simulink model "PassengerCar"  (R2019b)
settings: Solver=ode1  StartTime=0  StopTime=25  FixedStep=1.0000000000000000e-003  RelTol=1e-3
InitFcn:
  | sampleTime = str2double(get_param(bdroot, 'FixedStep'));
undefined symbols (not defined in the file or in its folder): AccPedalPos, BrakePedalPos, BrakeSwitch, DiscIntNeverNeededParam, DYNA4, EngSpd, IgnitionSwitch, InitialGear, InitialSpeed, IntendedEngTrq, LeftIndicator, MainBrakePress, MaxGear, MDL, MinGear, RefAcc, RefLane, RefLatPos, RefPath, RefPathCurv, RefSpd, RefSpdPreview, RefSpdRetrospect, RightIndicator, SteeringWheelAng, SteeringWheelTrq, UserDefinedRefValue, vm_const
libraries: UtilitiesLibrary x31, simulink x18, WheelSystemModules x13, LongitudinalControllerModules x13, LateralControllerModules x7, AnimationBusselectorModules x5, EnvironmentModules x5, BasicEngineControlModules x5, MiscellaneousControlModules x5, Animation3Modules x4, AuxiliariesModules x4, TireModules x4
(part 29 of 39)

== system PassengerCar/Vehicle/BrakeSystem/BrakeSystemControlUnit/BasicElectronicStabilityControl/BasicAntiLockBrakeControl ==
  ABSSwitchFromVehicleControl[0;1] : Inport
  RequiredWheelBrakePressures[Pa] : Inport  Port=2
  Vel_wrt_WorldSys(VehSys)[m/s] : Inport  Description=Maximum brake pressure  Port=3
  FrontLeftWheelLongSpd(ContactSys)[m/s] : Inport  Port=4
  FrontLeftWheelRotSpd[rad/s] : Inport  Port=5
  FrontLeftWheelRotAcc[rad/s**2] : Inport  Port=6
  FrontLeftTireDynamicRadius[m] : Inport  Port=7
  FrontRightWheelLongSpd(ContactSys)[m/s] : Inport  Port=8
  FrontRightWheelRotSpd[rad/s] : Inport  Port=9
  FrontRightWheelRotAcc[rad/s**2] : Inport  Port=10
  FrontRightTireDynamicRadius[m] : Inport  Port=11
  RearLeftWheelLongSpd(ContactSys)[m/s] : Inport  Port=12
  RearLeftWheelRotSpd[rad/s] : Inport  Port=13
  RearLeftWheelRotAcc[rad/s**2] : Inport  Port=14
  RearLeftTireDynamicRadius[m] : Inport  Port=15
  RearRightWheelLongSpd(ContactSys)[m/s] : Inport  Port=16
  RearRightWheelRotSpd[rad/s] : Inport  Port=17
  RearRightWheelRotAcc[rad/s**2] : Inport  Port=18
  RearRightTireDynamicRadius[m] : Inport  Port=19
  MaxMainBrakePress[Pa] : Inport  Description=Maximum brake pressure  Port=20
  AntiLockBrakeSystemOutput : Subsystem  Tag=TESIS DYNAware Interface Block  mask{NeedsUpdate=off, SignalInfo=|}
      mask SignalInfo=|
      | {
      |   "Version": "4.6",
      |   "MuxedOutputBusName": "AntiLockBrakeSystemInfo",
      |   "MuxedInputBusName": "input",
      |   "MuxedInputSelected": false,
      |   "MuxedOutputSelected": true,
      |   "SignalData": [
      |     {
      |       "initialValue": "0.0",
      |       "name": "FrontLeftWheelBrakeControllerState[0;3]",
      |       "comment": "",
      |       "minString": "",
      |       "maxString": "",
      |       "width": 1,
      |       "dataType": 0,
      |       "signalType": 0,
      |       "createSignal": false,
      |       "outputName": "FrontLeft.WheelBrakeControllerState[0;3]",
      |       "generateSignalAccessBlock": false,
      |       "accessId": "$(parentId).$(blockName).$(outputName)"
      |     },
      |     {
      |       "initialValue": "0.0",
      |       "name": "FrontRightWheelBrakeControllerState[0;3]",
      |       "comment": "",
      |       "minString": "",
      |       "maxString": "",
      |       "width": 1,
      |       "dataType": 0,
      |       "signalType": 0,
      |       "createSignal": false,
      |       "outputName": "FrontRight.WheelBrakeControllerState[0;3]",
      |       "generateSignalAccessBlock": false,
      |       "accessId": "$(parentId).$(blockName).$(outputName)"
      |     },
      |     {
      |       "initialValue": "0.0",
      |       "name": "RearLeftWheelBrakeControllerState[0;3]",
      |       "comment": "",
      |       "minString": "",
      |       "maxString": "",
      |       "width": 1,
      |       "dataType": 0,
      |       "signalType": 0,
      |       "createSignal": false,
      |       "outputName": "RearLeft.WheelBrakeControllerState[0;3]",
      |       "generateSignalAccessBlock": false,
      |       "accessId": "$(parentId).$(blockName).$(outputName)"
      |     },
      |     {
      |       "initialValue": "0.0",
      |       "name": "RearRightWheelBrakeControllerState[0;3]",
      |       "comment": "",
      |       "minString": "",
      |       "maxString": "",
      |       "width": 1,
      |       "dataType": 0,
      |       "signalType": 0,
      |       "createSignal": false,
      |       "outputName": "RearRight.WheelBrakeControllerState[0;3]",
      |       "generateSignalAccessBlock": false,
      |       "accessId": "$(parentId).$(blockName).$(outputName)"
      |     },
      |     {
      |       "initialValue": "0.0",
      |       "name": "FrontLeftAntiLockBrakeSystemActive[0;1]",
      |       "comment": "",
      |       "minString": "",
      |       "maxString": "",
      |       "width": 1,
      |       "dataType": 0,
      |       "signalType": 0,
      |       "createSignal": false,
      |       "outputName": "FrontLeft.AntiLockBrakeSystemActive[0;1]",
      |       "generateSignalAccessBlock": false,
      |       "accessId": "$(parentId).$(blockName).$(outputName)"
      |     },
      |     {
      |       "initialValue": "0.0",
      |       "name": "FrontRightAntiLockBrakeSystemActive[0;1]",
      |       "comment": "",
      |       "minString": "",
      |       "maxString": "",
      |       "width": 1,
      |       "dataType": 0,
      |       "signalType": 0,
      |       "createSignal": false,
      |       "outputName": "FrontRight.AntiLockBrakeSystemActive[0;1]",
      |       "generateSignalAccessBlock": false,
      |       "accessId": "$(parentId).$(blockName).$(outputName)"
      |     },
      |     {
      |       "initialValue": "0.0",
      |       "name": "RearLeftAntiLockBrakeSystemActive[0;1]",
      |       "comment": "",
      |       "minString": "",
      |       "maxString": "",
      |       "width": 1,
      |       "dataType": 0,
      |       "signalType": 0,
      |       "createSignal": false,
      |       "outputName": "RearLeft.AntiLockBrakeSystemActive[0;1]",
      |       "generateSignalAccessBlock": false,
      |       "accessId": "$(parentId).$(blockName).$(outputName)"
      |     },
      |     {
      |       "initialValue": "0.0",
      |       "name": "RearRightAntiLockBrakeSystemActive[0;1]",
      |       "comment": "",
      |       "minString": "",
      |       "maxString": "",
      |       "width": 1,
      |       "dataType": 0,
      |       "signalType": 0,
      |       "createSignal": false,
      |       "outputName": "RearRight.AntiLockBrakeSystemActive[0;1]",
      |       "generateSignalAccessBlock": false,
      |       "accessId": "$(parentId).$(blockName).$(outputName)"
      |     },
      |     {
      |       "initialValue": "0.0",
      |       "name": "Enabled[0;1]",
      |       "comment": "",
      |       "minString": "",
      |       "maxString": "",
      |       "width": 1,
      |       "dataType": 0,
      |       "signalType": 0,
      |       "createSignal": false,
      |       "outputName": "Enabled[0;1]",
      |       "generateSignalAccessBlock": false,
      |       "accessId": "$(parentId).$(blockName).$(outputName)"
      |     },
      |     {
      |       "initialValue": "0.0",
      |       "name": "Active[0;1]",
      |       "comment": "",
      |       "minString": "",
      |       "maxString": "",
      |       "width": 1,
      |       "dataType": 0,
      |       "signalType": 0,
      |       "createSignal": false,
      |       "outputName": "Active[0;1]",
      |       "generateSignalAccessBlock": false,
      |       "accessId": "$(parentId).$(blockName).$(outputName)"
      |     }
      |   ]
      | }
      mask prompts: NeedsUpdate "Specify, if subsystem content needs to be updated"; SignalInfo "Signal Info (json)"
      mask help: DYNA4 Interface Block Version 4.6
      mask init:
      | blockName = get_param(gcbh, 'Name');
      | parentId = DYNA4.ModelHandling.AccessID.getFromHierarchy(gcbh);
      | TD.InterfaceBlock.ModelCallbacks.GenerateContent(gcb);
      settings: DeleteFcn=TD.InterfaceBlock.ModelCallbacks.CloseGUI( gcbh );  NameChangeFcn=TD.InterfaceBlock.ModelCallbacks.BlockRenamedHandler(gcbh);  OpenFcn=TD.InterfaceBlock.ModelCallbacks.OpenGUI( gcbh );  CloseFcn=TD.InterfaceBlock.ModelCallbacks.CloseGUI( gcbh );
      mask Display:
      | image('InterfaceBlock.png','center');
      | port_label('input',1, 'FrontLeftWheelBrakeControllerState[0;3]');
      | port_label('input',2, 'FrontRightWheelBrakeControllerState[0;3]');
      | port_label('input',3, 'RearLeftWheelBrakeControllerState[0;3]');
      | port_label('input',4, 'RearRightWheelBrakeControllerState[0;3]');
      | port_label('input',5, 'FrontLeftAntiLockBrakeSystemActive[0;1]');
      | port_label('input',6, 'FrontRightAntiLockBrakeSystemActive[0;1]');
      | port_label('input',7, 'RearLeftAntiLockBrakeSystemActive[0;1]');
      | port_label('input',8, 'RearRightAntiLockBrakeSystemActive[0;1]');
      | port_label('input',9, 'Enabled[0;1]');
      | port_label('input',10, 'Active[0;1]');
      | port_label('output',1, 'AntiLockBrakeSystemInfo');
  BasicAntiLockBrakeSystem : BrakeSystemModules/BasicAntiLockBrakeSystem  DATA_NODE=MDL.Vehicle.BrakeSystem.BrakeSystemControlUnit.BasicAntiLockBrakeSystem  PressBuildupTimeConst=MDL.Vehicle.BrakeSystem.BrakeSystemControlUnit.BasicAntiLockBrakeSystem.PressBuildupTimeConst  RotDecelScaling=MDL.Vehicle.BrakeSystem.BrakeSystemControlUnit.BasicAntiLockBrakeSystem.RotDecelScaling  SlipScaling=MDL.Vehicle.BrakeSystem.BrakeSystemControlUnit.BasicAntiLockBrakeSystem.SlipScaling  UpperPressReductionThres=MDL.Vehicle.BrakeSystem.BrakeSystemControlUnit.BasicAntiLockBrakeSystem.SwitchCriteriaUpperThres  PressIncreaseLowerThres=MDL.Vehicle.BrakeSystem.BrakeSystemControlUnit.BasicAntiLockBrakeSystem.SwitchCriteriaLowerThres  PressIncreaseTimeConst=MDL.Vehicle.BrakeSystem.BrakeSystemControlUnit.BasicAntiLockBrakeSystem.PressIncreaseTimeConst  PressReductionTimeConst=MDL.Vehicle.BrakeSystem.BrakeSystemControlUnit.BasicAntiLockBrakeSystem.PressReductionTimeConst  LowerActivationSpdThres=MDL.Vehicle.BrakeSystem.BrakeSystemControlUnit.BasicAntiLockBrakeSystem.LowerActivationSpdThres  LowerActivationPressThres=MDL.Vehicle.BrakeSystem.BrakeSystemControlUnit.BasicAntiLockBrakeSystem.LowerActivationPressThres  Enable=MDL.Vehicle.BrakeSystem.BrakeSystemControlUnit.BasicAntiLockBrakeSystem.Enable
  Demux : Demux
  Mux : Mux
  WheelBrakePressures[Pa] : Outport  VectorParamsAs1DForOutWhenUnconnected=off
  Active[0;1] : Outport  Port=2  VectorParamsAs1DForOutWhenUnconnected=off
  AntiLockBrakeSystemInfo : Outport  Port=3  VectorParamsAs1DForOutWhenUnconnected=off
  wires:
  BasicAntiLockBrakeSystem/5 -> AntiLockBrakeSystemOutput/1(FrontLeftWheelBrakeControllerState[0;3]___UNIQUE_1)
  BasicAntiLockBrakeSystem/6 -> AntiLockBrakeSystemOutput/2(FrontRightWheelBrakeControllerState[0;3]___UNIQUE_1)
  BasicAntiLockBrakeSystem/12 -> AntiLockBrakeSystemOutput/8(RearRightAntiLockBrakeSystemActive[0;1]___UNIQUE_1)
  BasicAntiLockBrakeSystem/7 -> AntiLockBrakeSystemOutput/3(RearLeftWheelBrakeControllerState[0;3]___UNIQUE_1)
  BasicAntiLockBrakeSystem/11 -> AntiLockBrakeSystemOutput/7(RearLeftAntiLockBrakeSystemActive[0;1]___UNIQUE_1)
  BasicAntiLockBrakeSystem/8 -> AntiLockBrakeSystemOutput/4(RearRightWheelBrakeControllerState[0;3]___UNIQUE_1)
  BasicAntiLockBrakeSystem/10 -> AntiLockBrakeSystemOutput/6(FrontRightAntiLockBrakeSystemActive[0;1]___UNIQUE_1)
  BasicAntiLockBrakeSystem/9 -> AntiLockBrakeSystemOutput/5(FrontLeftAntiLockBrakeSystemActive[0;1]___UNIQUE_1)
  AntiLockBrakeSystemOutput/1(AntiLockBrakeSystemInfo___UNIQUE_1) -> AntiLockBrakeSystemInfo/1
  Mux/1 -> WheelBrakePressures[Pa]/1
  BasicAntiLockBrakeSystem/4 -> Mux/4
  BasicAntiLockBrakeSystem/3 -> Mux/3
  BasicAntiLockBrakeSystem/2 -> Mux/2
  BasicAntiLockBrakeSystem/1 -> Mux/1
  Vel_wrt_WorldSys(VehSys)[m/s]/1 -> BasicAntiLockBrakeSystem/2
  Demux/1 -> BasicAntiLockBrakeSystem/20
  Demux/2 -> BasicAntiLockBrakeSystem/21
  Demux/3 -> BasicAntiLockBrakeSystem/22
  MaxMainBrakePress[Pa]/1 -> BasicAntiLockBrakeSystem/19
  Demux/4 -> BasicAntiLockBrakeSystem/23
  ABSSwitchFromVehicleControl[0;1]/1 -> BasicAntiLockBrakeSystem/1
  FrontRightWheelRotAcc[rad/s**2]/1 -> BasicAntiLockBrakeSystem/9
  RearLeftTireDynamicRadius[m]/1 -> BasicAntiLockBrakeSystem/14
  FrontLeftWheelLongSpd(ContactSys)[m/s]/1 -> BasicAntiLockBrakeSystem/3
  RearRightWheelRotSpd[rad/s]/1 -> BasicAntiLockBrakeSystem/16
  FrontLeftWheelRotSpd[rad/s]/1 -> BasicAntiLockBrakeSystem/4
  FrontRightTireDynamicRadius[m]/1 -> BasicAntiLockBrakeSystem/10
  RearRightTireDynamicRadius[m]/1 -> BasicAntiLockBrakeSystem/18
  FrontLeftWheelRotAcc[rad/s**2]/1 -> BasicAntiLockBrakeSystem/5
  RearRightWheelRotAcc[rad/s**2]/1 -> BasicAntiLockBrakeSystem/17
  RearRightWheelLongSpd(ContactSys)[m/s]/1 -> BasicAntiLockBrakeSystem/15
  RearLeftWheelRotAcc[rad/s**2]/1 -> BasicAntiLockBrakeSystem/13
  FrontLeftTireDynamicRadius[m]/1 -> BasicAntiLockBrakeSystem/6
  RearLeftWheelRotSpd[rad/s]/1 -> BasicAntiLockBrakeSystem/12
  FrontRightWheelRotSpd[rad/s]/1 -> BasicAntiLockBrakeSystem/8
  RearLeftWheelLongSpd(ContactSys)[m/s]/1 -> BasicAntiLockBrakeSystem/11
  FrontRightWheelLongSpd(ContactSys)[m/s]/1 -> BasicAntiLockBrakeSystem/7
  RequiredWheelBrakePressures[Pa]/1 -> Demux/1
  BasicAntiLockBrakeSystem/13 -> AntiLockBrakeSystemOutput/9(Enabled[0;1]___UNIQUE_1)
  BasicAntiLockBrakeSystem/14 -> Active[0;1]/1, AntiLockBrakeSystemOutput/10(Active[0;1]___UNIQUE_1)

== system PassengerCar/Vehicle/BrakeSystem/BrakeSystemControlUnit/BasicElectronicStabilityControl/BasicYawStabilityControl ==
  ESCSwitch[0;1] : Inport
  WheelBrakePressureFromBrakeHydraulics : Inport  Port=2
  Vel_wrt_WorldSys(VehSys)[m/s] : Inport  Port=3
  Acc_wrt_WorldSys(VehSys)[m/**s2] : Inport  Port=4
  YawRate[rad/s] : Inport  Port=5
  YawInertia[kgm2] : Inport  Port=6
  FrontWheelTrack[m] : Inport  Port=7
  RearWheelTrack[m] : Inport  Port=8
  FrontLeftTireRadius[m] : Inport  Port=9
  RearLeftTireRadius[m] : Inport  Port=10
  FrontBrakeTrqPressRatio[m**3] : Inport  Port=11
  RearBrakeTrqPressRatio[m**3] : Inport  Port=12
  BasicYawStabilityControl : BrakeSystemModules/BasicYawStabilityControl  DATA_NODE=MDL.Vehicle.BrakeSystem.BrakeSystemControlUnit.BasicYawStabilityControl  Vehicle=MDL.Vehicle.BrakeSystem.BrakeSystemControlUnit.BasicYawStabilityControl.Vehicle  Control=MDL.Vehicle.BrakeSystem.BrakeSystemControlUnit.BasicYawStabilityControl.Control  Enable=MDL.Vehicle.BrakeSystem.BrakeSystemControlUnit.BasicYawStabilityControl.Enable
  Mux : Mux
  PrepareBrakeTrqPressRatioInput : Subsystem
  PrepareTireRadiusInput : Subsystem
  PrepareWheelTrackInput : Subsystem
  Selector : Selector  InputPortWidth=3  IndexOptions=Index vector (dialog)  Indices=1  OutputSizes=1
  Selector1 : Selector  InputPortWidth=3  IndexOptions=Index vector (dialog)  Indices=2  OutputSizes=1
  YawStabilityControlOutput : Subsystem  Tag=TESIS DYNAware Interface Block  mask{NeedsUpdate=off, SignalInfo=|}
      mask SignalInfo=|
      | {
      |   "Version": "4.6",
      |   "MuxedOutputBusName": "YawStabilityControlInfo",
      |   "MuxedInputBusName": "input",
      |   "MuxedInputSelected": false,
      |   "MuxedOutputSelected": true,
      |   "SignalData": [
      |     {
      |       "initialValue": "0.0",
      |       "name": "Active[0;1]",
      |       "comment": "",
      |       "minString": "",
      |       "maxString": "",
      |       "width": 1,
      |       "dataType": 0,
      |       "signalType": 0,
      |       "createSignal": false,
      |       "outputName": "Active[0;1]",
      |       "generateSignalAccessBlock": false,
      |       "accessId": "$(parentId).$(blockName).$(outputName)"
      |     },
      |     {
      |       "initialValue": "0.0",
      |       "name": "Enabled[0;1]",
      |       "comment": "",
      |       "minString": "",
      |       "maxString": "",
      |       "width": 1,
      |       "dataType": 0,
      |       "signalType": 0,
      |       "createSignal": false,
      |       "outputName": "Enabled[0;1]",
      |       "generateSignalAccessBlock": false,
      |       "accessId": "$(parentId).$(blockName).$(outputName)"
      |     }
      |   ]
      | }
      mask prompts: NeedsUpdate "Specify, if subsystem content needs to be updated"; SignalInfo "Signal Info (json)"
      mask help: DYNA4 Interface Block Version 4.6
      mask init:
      | blockName = get_param(gcbh, 'Name');
      | parentId = DYNA4.ModelHandling.AccessID.getFromHierarchy(gcbh);
      | TD.InterfaceBlock.ModelCallbacks.GenerateContent(gcb);
      settings: DeleteFcn=TD.InterfaceBlock.ModelCallbacks.CloseGUI( gcbh );  NameChangeFcn=TD.InterfaceBlock.ModelCallbacks.BlockRenamedHandler(gcbh);  OpenFcn=TD.InterfaceBlock.ModelCallbacks.OpenGUI( gcbh );  CloseFcn=TD.InterfaceBlock.ModelCallbacks.CloseGUI( gcbh );
      mask Display:
      | image('InterfaceBlock.png','center');
      | port_label('input',1, 'Active[0;1]');
      | port_label('input',2, 'Enabled[0;1]');
      | port_label('output',1, 'YawStabilityControlInfo');
  WheelBrakePressures[Pa] : Outport  VectorParamsAs1DForOutWhenUnconnected=off
  Active[0;1] : Outport  Port=2  VectorParamsAs1DForOutWhenUnconnected=off
  YawStabilityControlInfo : Outport  Port=3  VectorParamsAs1DForOutWhenUnconnected=off
  wires:
  BasicYawStabilityControl/5 -> Mux/4
  Mux/1 -> WheelBrakePressures[Pa]/1
  Selector1/1 -> BasicYawStabilityControl/3
  PrepareBrakeTrqPressRatioInput/1(AverageBrakeTrqPressRatio[m**3]) -> BasicYawStabilityControl/8
  PrepareTireRadiusInput/1(AverageTireRadius[m]) -> BasicYawStabilityControl/7
  FrontBrakeTrqPressRatio[m**3]/1 -> PrepareBrakeTrqPressRatioInput/1(FrontBrakeTrqPressRatio[m**3])
  BasicYawStabilityControl/1 -> YawStabilityControlOutput/1(Active[0;1]___UNIQUE_1), Active[0;1]/1
  RearBrakeTrqPressRatio[m**3]/1 -> PrepareBrakeTrqPressRatioInput/2(RearBrakeTrqPressRatio[m**3])
  BasicYawStabilityControl/2 -> Mux/1
  BasicYawStabilityControl/4 -> Mux/3
  BasicYawStabilityControl/3 -> Mux/2
  Selector/1 -> BasicYawStabilityControl/2
  RearWheelTrack[m]/1 -> PrepareWheelTrackInput/2(RearWheelTrack[m])
  FrontWheelTrack[m]/1 -> PrepareWheelTrackInput/1(FrontWheelTrack[m])
  FrontLeftTireRadius[m]/1 -> PrepareTireRadiusInput/1(FrontLeftTireRadius[m])
  PrepareWheelTrackInput/1(AverageWheelTrack[m]) -> BasicYawStabilityControl/6
  RearLeftTireRadius[m]/1 -> PrepareTireRadiusInput/2(RearLeftTireRadius[m])
  Acc_wrt_WorldSys(VehSys)[m/**s2]/1 -> Selector1/1
  Vel_wrt_WorldSys(VehSys)[m/s]/1 -> Selector/1
  ESCSwitch[0;1]/1 -> BasicYawStabilityControl/1
  YawInertia[kgm2]/1 -> BasicYawStabilityControl/5
  YawRate[rad/s]/1 -> BasicYawStabilityControl/4
  WheelBrakePressureFromBrakeHydraulics/1 -> BasicYawStabilityControl/9
  BasicYawStabilityControl/6 -> YawStabilityControlOutput/2(Enabled[0;1]___UNIQUE_1)
  YawStabilityControlOutput/1(YawStabilityControlInfo___UNIQUE_1) -> YawStabilityControlInfo/1

== system PassengerCar/Vehicle/BrakeSystem/BrakeSystemControlUnit/BasicElectronicStabilityControlInput/InputFromBrakeSystemPhysics ==
  fromBrakeSystemPhysics : Inport
  TDBusSelector : BusSelector  OutputSignals=MaxMainBrakePress[Pa],FrontLeftWheelBrakePress[Pa],FrontRightWheelBrakePress[Pa],RearLeftWheelBrakePress[Pa],RearRightWheelBrakePress[Pa]
  __TDD__FrontLeftWheelBrakePress[Pa] : Demux  Outputs=1
  __TDD__FrontRightWheelBrakePress[Pa] : Demux  Outputs=1
  __TDD__MaxMainBrakePress[Pa] : Demux  Outputs=1
  __TDD__RearLeftWheelBrakePress[Pa] : Demux  Outputs=1
  __TDD__RearRightWheelBrakePress[Pa] : Demux  Outputs=1
  MaxMainBrakePress[Pa]___UNIQUE_1 : Outport  Description=|  VectorParamsAs1DForOutWhenUnconnected=off
      | <name>MaxMainBrakePress[Pa]</name>
      | <comment></comment>
  FrontLeftWheelBrakePress[Pa]___UNIQUE_1 : Outport  Description=|  Port=2  VectorParamsAs1DForOutWhenUnconnected=off
      | <name>FrontLeftWheelBrakePress[Pa]</name>
      | <comment></comment>
  FrontRightWheelBrakePress[Pa]___UNIQUE_1 : Outport  Description=|  Port=3  VectorParamsAs1DForOutWhenUnconnected=off
      | <name>FrontRightWheelBrakePress[Pa]</name>
      | <comment></comment>
  RearLeftWheelBrakePress[Pa]___UNIQUE_1 : Outport  Description=|  Port=4  VectorParamsAs1DForOutWhenUnconnected=off
      | <name>RearLeftWheelBrakePress[Pa]</name>
      | <comment></comment>
  RearRightWheelBrakePress[Pa]___UNIQUE_1 : Outport  Description=|  Port=5  VectorParamsAs1DForOutWhenUnconnected=off
      | <name>RearRightWheelBrakePress[Pa]</name>
      | <comment></comment>
  wires:
  fromBrakeSystemPhysics/1 -> TDBusSelector/1
  TDBusSelector/1 -> __TDD__MaxMainBrakePress[Pa]/1  "<MaxMainBrakePress[Pa]>"
  TDBusSelector/2 -> __TDD__FrontLeftWheelBrakePress[Pa]/1  "<FrontLeftWheelBrakePress[Pa]>"
  TDBusSelector/3 -> __TDD__FrontRightWheelBrakePress[Pa]/1  "<FrontRightWheelBrakePress[Pa]>"
  TDBusSelector/4 -> __TDD__RearLeftWheelBrakePress[Pa]/1  "<RearLeftWheelBrakePress[Pa]>"
  TDBusSelector/5 -> __TDD__RearRightWheelBrakePress[Pa]/1  "<RearRightWheelBrakePress[Pa]>"
  __TDD__MaxMainBrakePress[Pa]/1 -> MaxMainBrakePress[Pa]___UNIQUE_1/1  "MaxMainBrakePress[Pa]"
  __TDD__FrontLeftWheelBrakePress[Pa]/1 -> FrontLeftWheelBrakePress[Pa]___UNIQUE_1/1  "FrontLeftWheelBrakePress[Pa]"
  __TDD__FrontRightWheelBrakePress[Pa]/1 -> FrontRightWheelBrakePress[Pa]___UNIQUE_1/1  "FrontRightWheelBrakePress[Pa]"
  __TDD__RearLeftWheelBrakePress[Pa]/1 -> RearLeftWheelBrakePress[Pa]___UNIQUE_1/1  "RearLeftWheelBrakePress[Pa]"
  __TDD__RearRightWheelBrakePress[Pa]/1 -> RearRightWheelBrakePress[Pa]___UNIQUE_1/1  "RearRightWheelBrakePress[Pa]"

== system PassengerCar/Vehicle/BrakeSystem/BrakeSystemControlUnit/BasicElectronicStabilityControlInput/InputFromCTRL ==
  fromCTRL : Inport
  TDBusSelector : BusSelector  OutputSignals=CTRL.LongitudinalControl.ABSSwitch[0;1],CTRL.LongitudinalControl.ESCSwitch[0;1]
  __TDD__ABSSwitch[0;1] : Demux  Outputs=[1]
  __TDD__ESCSwitch[0;1] : Demux  Outputs=[1]
  ABSSwitch[0;1]___UNIQUE_1 : Outport  Description=|  PortDimensions=[1]  VectorParamsAs1DForOutWhenUnconnected=off
      | <name>CTRL.LongitudinalControl.ABSSwitch[0;1]</name>
      | <comment></comment>
  ESCSwitch[0;1]___UNIQUE_1 : Outport  Description=|  Port=2  PortDimensions=[1]  VectorParamsAs1DForOutWhenUnconnected=off
      | <name>CTRL.LongitudinalControl.ESCSwitch[0;1]</name>
      | <comment></comment>
  wires:
  fromCTRL/1 -> TDBusSelector/1
  TDBusSelector/1 -> __TDD__ABSSwitch[0;1]/1  "<ABSSwitch[0;1]>"
  TDBusSelector/2 -> __TDD__ESCSwitch[0;1]/1  "<ESCSwitch[0;1]>"
  __TDD__ABSSwitch[0;1]/1 -> ABSSwitch[0;1]___UNIQUE_1/1  "ABSSwitch[0;1]"
  __TDD__ESCSwitch[0;1]/1 -> ESCSwitch[0;1]___UNIQUE_1/1  "ESCSwitch[0;1]"

== system PassengerCar/Vehicle/BrakeSystem/BrakeSystemControlUnit/BasicElectronicStabilityControlInput/InputFromChassis ==
  fromChassis : Inport
  TDBusSelector : BusSelector  OutputSignals=VehicleBody.Vel_wrt_WorldSys(VehSys)[m/s],VehicleBody.Acc_wrt_WorldSys(VehSys)[m/s**2],VehicleBody.YawRate[rad/s],VehicleBody.CoGYawInrt(VehSys)[kg*m**2],FrontAxle.WheelTrack[m],RearAxle.WheelTrack[m]
  __TDD__Acc_wrt_WorldSys(VehSys)[m/s**2] : Demux  Outputs=[3]
  __TDD__CoGYawInrt(VehSys)[kg*m**2] : Demux  Outputs=[1]
  __TDD__RearWheelTrack[m] : Demux  Outputs=[1]
  __TDD__Vel_wrt_WorldSys(VehSys)[m/s] : Demux  Outputs=[3]
  __TDD__WheelTrack[m] : Demux  Outputs=[1]
  __TDD__YawRate[rad/s] : Demux  Outputs=[1]
  Vel_wrt_WorldSys(VehSys)[m/s]___UNIQUE_1 : Outport  Description=|  PortDimensions=[3]  VectorParamsAs1DForOutWhenUnconnected=off
      | <name>VehicleBody.Vel_wrt_WorldSys(VehSys)[m/s]</name>
      | <comment></comment>
  Acc_wrt_WorldSys(VehSys)[m/s**2]___UNIQUE_1 : Outport  Description=|  Port=2  PortDimensions=[3]  VectorParamsAs1DForOutWhenUnconnected=off
      | <name>VehicleBody.Acc_wrt_WorldSys(VehSys)[m/s**2]</name>
      | <comment></comment>
  YawRate[rad/s]___UNIQUE_1 : Outport  Description=|  Port=3  PortDimensions=[1]  VectorParamsAs1DForOutWhenUnconnected=off
      | <name>VehicleBody.YawRate[rad/s]</name>
      | <comment></comment>
  CoGYawInrt(VehSys)[kg*m**2]___UNIQUE_1 : Outport  Description=|  Port=4  PortDimensions=[1]  VectorParamsAs1DForOutWhenUnconnected=off
      | <name>VehicleBody.CoGYawInrt(VehSys)[kg*m**2]</name>
      | <comment></comment>
  WheelTrack[m]___UNIQUE_1 : Outport  Description=|  Port=5  PortDimensions=[1]  VectorParamsAs1DForOutWhenUnconnected=off
      | <name>FrontAxle.WheelTrack[m]</name>
      | <comment></comment>
  RearWheelTrack[m]___UNIQUE_1 : Outport  Description=|  Port=6  PortDimensions=[1]  VectorParamsAs1DForOutWhenUnconnected=off
      | <name>RearAxle.WheelTrack[m]</name>
      | <comment></comment>
  wires:
  fromChassis/1 -> TDBusSelector/1
  TDBusSelector/1 -> __TDD__Vel_wrt_WorldSys(VehSys)[m/s]/1  "<Vel_wrt_WorldSys(VehSys)[m/s]>"
  TDBusSelector/2 -> __TDD__Acc_wrt_WorldSys(VehSys)[m/s**2]/1  "<Acc_wrt_WorldSys(VehSys)[m/s**2]>"
  TDBusSelector/3 -> __TDD__YawRate[rad/s]/1  "<YawRate[rad/s]>"
  TDBusSelector/4 -> __TDD__CoGYawInrt(VehSys)[kg*m**2]/1  "<CoGYawInrt(VehSys)[kg*m**2]>"
  TDBusSelector/5 -> __TDD__WheelTrack[m]/1  "<WheelTrack[m]>"
  TDBusSelector/6 -> __TDD__RearWheelTrack[m]/1  "<WheelTrack[m]>"
  __TDD__Vel_wrt_WorldSys(VehSys)[m/s]/1 -> Vel_wrt_WorldSys(VehSys)[m/s]___UNIQUE_1/1  "Vel_wrt_WorldSys(VehSys)[m/s]"
  __TDD__Acc_wrt_WorldSys(VehSys)[m/s**2]/1 -> Acc_wrt_WorldSys(VehSys)[m/s**2]___UNIQUE_1/1  "Acc_wrt_WorldSys(VehSys)[m/s**2]"
  __TDD__YawRate[rad/s]/1 -> YawRate[rad/s]___UNIQUE_1/1  "YawRate[rad/s]"
  __TDD__CoGYawInrt(VehSys)[kg*m**2]/1 -> CoGYawInrt(VehSys)[kg*m**2]___UNIQUE_1/1  "CoGYawInrt(VehSys)[kg*m**2]"
  __TDD__WheelTrack[m]/1 -> WheelTrack[m]___UNIQUE_1/1  "WheelTrack[m]"
  __TDD__RearWheelTrack[m]/1 -> RearWheelTrack[m]___UNIQUE_1/1  "RearWheelTrack[m]"

== system PassengerCar/Vehicle/BrakeSystem/BrakeSystemControlUnit/BasicElectronicStabilityControlInput/InputFromWheelSystem ==
  fromWheelSystem : Inport
  TDBusSelector : BusSelector  OutputSignals=FrontLeft.Tire.LongSpd(ContactSys)[m/s],FrontLeft.Wheel.RotSpd[rad/s],FrontLeft.Wheel.RotAcc[rad/s**2],FrontLeft.Tire.DynamicRadius[m],FrontRight.Tire.LongSpd(ContactSys)[m/s],FrontRight.Wheel.RotSpd[rad/s],FrontRight.Wheel.RotAcc[rad/s**2],FrontRight.Tire.DynamicRadius[m],RearLeft.Tire.LongSpd(ContactSys)[m/s],RearLeft.Wheel.RotSpd[rad/s],RearLeft.Wheel.RotAcc[rad/s**2],RearLeft.Tire.DynamicRadius[m],RearRight.Tire.LongSpd(ContactSys)[m/s],RearRight.Wheel.RotSpd[rad/s],RearRight.Wheel.RotAcc[rad/s**2],RearRight.Tire.DynamicRadius[m],FrontLeft.Tire.UnloadedRadius[m],RearLeft.Tire.UnloadedRadius[m],FrontLeft.Wheel.BrakeTrqPressRatio[m**3],RearLeft.Wheel.BrakeTrqPressRatio[m**3]
  __TDD__FrontLeft_Tire_DynamicRadius[m] : Demux  Outputs=[1]
  __TDD__FrontLeft_Tire_LongSpd(ContactSys)[m/s] : Demux  Outputs=[1]
  __TDD__FrontLeft_Tire_UnloadedRadius[m] : Demux  Outputs=[1]
  __TDD__FrontLeft_Wheel_BrakeTrqPressRatio[m**3] : Demux  Outputs=[1]
  __TDD__FrontLeft_Wheel_RotAcc[rad/s**2] : Demux  Outputs=[1]
  __TDD__FrontLeft_Wheel_RotSpd[rad/s] : Demux  Outputs=1
  __TDD__FrontRight_Tire_DynamicRadius[m] : Demux  Outputs=[1]
  __TDD__FrontRight_Tire_LongSpd(ContactSys)[m/s] : Demux  Outputs=[1]
  __TDD__FrontRight_Wheel_RotAcc[rad/s**2] : Demux  Outputs=[1]
  __TDD__FrontRight_Wheel_RotSpd[rad/s] : Demux  Outputs=[1]
  __TDD__RearLeft_Tire_DynamicRadius[m] : Demux  Outputs=[1]
  __TDD__RearLeft_Tire_LongSpd(ContactSys)[m/s] : Demux  Outputs=[1]
  __TDD__RearLeft_Tire_UnloadedRadius[m] : Demux  Outputs=[1]
  __TDD__RearLeft_Wheel_BrakeTrqPressRatio[m**3] : Demux  Outputs=[1]
  __TDD__RearLeft_Wheel_RotAcc[rad/s**2] : Demux  Outputs=[1]
  __TDD__RearLeft_Wheel_RotSpd[rad/s] : Demux  Outputs=[1]
  __TDD__RearRight_Tire_DynamicRadius[m] : Demux  Outputs=[1]
  __TDD__RearRight_Tire_LongSpd(ContactSys)[m/s] : Demux  Outputs=[1]
  __TDD__RearRight_Wheel_RotAcc[rad/s**2] : Demux  Outputs=[1]
  __TDD__RearRight_Wheel_RotSpd[rad/s] : Demux  Outputs=[1]
  FrontLeft_Tire_LongSpd(ContactSys)[m/s]___UNIQUE_1 : Outport  Description=|  PortDimensions=[1]  VectorParamsAs1DForOutWhenUnconnected=off
      | <name>FrontLeft.Tire.LongSpd(ContactSys)[m/s]</name>
      | <comment>Front left longitudinal wheel speed in contact system</comment>
  FrontLeft_Wheel_RotSpd[rad/s]___UNIQUE_1 : Outport  Description=|  Port=2  VectorParamsAs1DForOutWhenUnconnected=off
      | <name>FrontLeft.Wheel.RotSpd[rad/s]</name>
      | <comment>Front left wheel rotational speed</comment>
  FrontLeft_Wheel_RotAcc[rad/s**2]___UNIQUE_1 : Outport  Description=|  Port=3  PortDimensions=[1]  VectorParamsAs1DForOutWhenUnconnected=off
      | <name>FrontLeft.Wheel.RotAcc[rad/s**2]</name>
      | <comment>Front left wheel rotational acceleration</comment>
  FrontLeft_Tire_DynamicRadius[m]___UNIQUE_1 : Outport  Description=|  Port=4  PortDimensions=[1]  VectorParamsAs1DForOutWhenUnconnected=off
      | <name>FrontLeft.Tire.DynamicRadius[m]</name>
      | <comment>Front left tire dynamic radius</comment>
  FrontRight_Tire_LongSpd(ContactSys)[m/s]___UNIQUE_1 : Outport  Description=|  Port=5  PortDimensions=[1]  VectorParamsAs1DForOutWhenUnconnected=off
      | <name>FrontRight.Tire.LongSpd(ContactSys)[m/s]</name>
      | <comment>Front right wheel longitudinal speed in contact system</comment>
  FrontRight_Wheel_RotSpd[rad/s]___UNIQUE_1 : Outport  Description=|  Port=6  PortDimensions=[1]  VectorParamsAs1DForOutWhenUnconnected=off
      | <name>FrontRight.Wheel.RotSpd[rad/s]</name>
      | <comment>Front right wheel rotational speed</comment>
  FrontRight_Wheel_RotAcc[rad/s**2]___UNIQUE_1 : Outport  Description=|  Port=7  PortDimensions=[1]  VectorParamsAs1DForOutWhenUnconnected=off
      | <name>FrontRight.Wheel.RotAcc[rad/s**2]</name>
      | <comment>Front right wheel rotational acceleration</comment>
  FrontRight_Tire_DynamicRadius[m]___UNIQUE_1 : Outport  Description=|  Port=8  PortDimensions=[1]  VectorParamsAs1DForOutWhenUnconnected=off
      | <name>FrontRight.Tire.DynamicRadius[m]</name>
      | <comment>Front right tire dynamic radius</comment>
  RearLeft_Tire_LongSpd(ContactSys)[m/s]___UNIQUE_1 : Outport  Description=|  Port=9  PortDimensions=[1]  VectorParamsAs1DForOutWhenUnconnected=off
      | <name>RearLeft.Tire.LongSpd(ContactSys)[m/s]</name>
      | <comment>Rear left wheel longitudinal speed in contact system</comment>
  RearLeft_Wheel_RotSpd[rad/s]___UNIQUE_1 : Outport  Description=|  Port=10  PortDimensions=[1]  VectorParamsAs1DForOutWhenUnconnected=off
      | <name>RearLeft.Wheel.RotSpd[rad/s]</name>
      | <comment>Rear left wheel rotational speed</comment>
  RearLeft_Wheel_RotAcc[rad/s**2]___UNIQUE_1 : Outport  Description=|  Port=11  PortDimensions=[1]  VectorParamsAs1DForOutWhenUnconnected=off
      | <name>RearLeft.Wheel.RotAcc[rad/s**2]</name>
      | <comment>Rear left wheel rotational acceleration</comment>
  RearLeft_Tire_DynamicRadius[m]___UNIQUE_1 : Outport  Description=|  Port=12  PortDimensions=[1]  VectorParamsAs1DForOutWhenUnconnected=off
      | <name>RearLeft.Tire.DynamicRadius[m]</name>
      | <comment>Rear left tire dynamic radius</comment>
  RearRight_Tire_LongSpd(ContactSys)[m/s]___UNIQUE_1 : Outport  Description=|  Port=13  PortDimensions=[1]  VectorParamsAs1DForOutWhenUnconnected=off
      | <name>RearRight.Tire.LongSpd(ContactSys)[m/s]</name>
      | <comment>Rear right wheel longitudinal speed in contact system</comment>
  RearRight_Wheel_RotSpd[rad/s]___UNIQUE_1 : Outport  Description=|  Port=14  PortDimensions=[1]  VectorParamsAs1DForOutWhenUnconnected=off
      | <name>RearRight.Wheel.RotSpd[rad/s]</name>
      | <comment>Rear right wheel rotational speed</comment>
  RearRight_Wheel_RotAcc[rad/s**2]___UNIQUE_1 : Outport  Description=|  Port=15  PortDimensions=[1]  VectorParamsAs1DForOutWhenUnconnected=off
      | <name>RearRight.Wheel.RotAcc[rad/s**2]</name>
      | <comment>Rear right wheel rotational acceleration</comment>
  RearRight_Tire_DynamicRadius[m]___UNIQUE_1 : Outport  Description=|  Port=16  PortDimensions=[1]  VectorParamsAs1DForOutWhenUnconnected=off
      | <name>RearRight.Tire.DynamicRadius[m]</name>
      | <comment>Rear right tire dynamic radius</comment>
  FrontLeft_Tire_UnloadedRadius[m]___UNIQUE_1 : Outport  Description=|  Port=17  PortDimensions=[1]  VectorParamsAs1DForOutWhenUnconnected=off
      | <name>FrontLeft.Tire.UnloadedRadius[m]</name>
      | <comment></comment>
  RearLeft_Tire_UnloadedRadius[m]___UNIQUE_1 : Outport  Description=|  Port=18  PortDimensions=[1]  VectorParamsAs1DForOutWhenUnconnected=off
      | <name>RearLeft.Tire.UnloadedRadius[m]</name>
      | <comment></comment>
  FrontLeft_Wheel_BrakeTrqPressRatio[m**3]___UNIQUE_1 : Outport  Description=|  Port=19  PortDimensions=[1]  VectorParamsAs1DForOutWhenUnconnected=off
      | <name>FrontLeft.Wheel.BrakeTrqPressRatio[m**3]</name>
      | <comment></comment>
  RearLeft_Wheel_BrakeTrqPressRatio[m**3]___UNIQUE_1 : Outport  Description=|  Port=20  PortDimensions=[1]  VectorParamsAs1DForOutWhenUnconnected=off
      | <name>RearLeft.Wheel.BrakeTrqPressRatio[m**3]</name>
      | <comment></comment>
  wires:
  fromWheelSystem/1 -> TDBusSelector/1
  TDBusSelector/1 -> __TDD__FrontLeft_Tire_LongSpd(ContactSys)[m/s]/1  "<LongSpd(ContactSys)[m/s]>"
  TDBusSelector/2 -> __TDD__FrontLeft_Wheel_RotSpd[rad/s]/1  "<RotSpd[rad/s]>"
  TDBusSelector/3 -> __TDD__FrontLeft_Wheel_RotAcc[rad/s**2]/1  "<RotAcc[rad/s**2]>"
  TDBusSelector/4 -> __TDD__FrontLeft_Tire_DynamicRadius[m]/1  "<DynamicRadius[m]>"
  TDBusSelector/5 -> __TDD__FrontRight_Tire_LongSpd(ContactSys)[m/s]/1  "<LongSpd(ContactSys)[m/s]>"
  TDBusSelector/6 -> __TDD__FrontRight_Wheel_RotSpd[rad/s]/1  "<RotSpd[rad/s]>"
  TDBusSelector/7 -> __TDD__FrontRight_Wheel_RotAcc[rad/s**2]/1  "<RotAcc[rad/s**2]>"
  TDBusSelector/8 -> __TDD__FrontRight_Tire_DynamicRadius[m]/1  "<DynamicRadius[m]>"
  TDBusSelector/9 -> __TDD__RearLeft_Tire_LongSpd(ContactSys)[m/s]/1  "<LongSpd(ContactSys)[m/s]>"
  TDBusSelector/10 -> __TDD__RearLeft_Wheel_RotSpd[rad/s]/1  "<RotSpd[rad/s]>"
  TDBusSelector/11 -> __TDD__RearLeft_Wheel_RotAcc[rad/s**2]/1  "<RotAcc[rad/s**2]>"
  TDBusSelector/12 -> __TDD__RearLeft_Tire_DynamicRadius[m]/1  "<DynamicRadius[m]>"
  TDBusSelector/13 -> __TDD__RearRight_Tire_LongSpd(ContactSys)[m/s]/1  "<LongSpd(ContactSys)[m/s]>"
  TDBusSelector/14 -> __TDD__RearRight_Wheel_RotSpd[rad/s]/1  "<RotSpd[rad/s]>"
  TDBusSelector/15 -> __TDD__RearRight_Wheel_RotAcc[rad/s**2]/1  "<RotAcc[rad/s**2]>"
  TDBusSelector/16 -> __TDD__RearRight_Tire_DynamicRadius[m]/1  "<DynamicRadius[m]>"
  TDBusSelector/17 -> __TDD__FrontLeft_Tire_UnloadedRadius[m]/1  "<UnloadedRadius[m]>"
  TDBusSelector/18 -> __TDD__RearLeft_Tire_UnloadedRadius[m]/1  "<UnloadedRadius[m]>"
  TDBusSelector/19 -> __TDD__FrontLeft_Wheel_BrakeTrqPressRatio[m**3]/1  "<BrakeTrqPressRatio[m**3]>"
  TDBusSelector/20 -> __TDD__RearLeft_Wheel_BrakeTrqPressRatio[m**3]/1  "<BrakeTrqPressRatio[m**3]>"
  __TDD__FrontLeft_Tire_LongSpd(ContactSys)[m/s]/1 -> FrontLeft_Tire_LongSpd(ContactSys)[m/s]___UNIQUE_1/1  "FrontLeft_Tire_LongSpd(ContactSys)[m/s]"
  __TDD__FrontLeft_Wheel_RotSpd[rad/s]/1 -> FrontLeft_Wheel_RotSpd[rad/s]___UNIQUE_1/1  "FrontLeft_Wheel_RotSpd[rad/s]"
  __TDD__FrontLeft_Wheel_RotAcc[rad/s**2]/1 -> FrontLeft_Wheel_RotAcc[rad/s**2]___UNIQUE_1/1  "FrontLeft_Wheel_RotAcc[rad/s**2]"
  __TDD__FrontLeft_Tire_DynamicRadius[m]/1 -> FrontLeft_Tire_DynamicRadius[m]___UNIQUE_1/1  "FrontLeft_Tire_DynamicRadius[m]"
  __TDD__FrontRight_Tire_LongSpd(ContactSys)[m/s]/1 -> FrontRight_Tire_LongSpd(ContactSys)[m/s]___UNIQUE_1/1  "FrontRight_Tire_LongSpd(ContactSys)[m/s]"
  __TDD__FrontRight_Wheel_RotSpd[rad/s]/1 -> FrontRight_Wheel_RotSpd[rad/s]___UNIQUE_1/1  "FrontRight_Wheel_RotSpd[rad/s]"
  __TDD__FrontRight_Wheel_RotAcc[rad/s**2]/1 -> FrontRight_Wheel_RotAcc[rad/s**2]___UNIQUE_1/1  "FrontRight_Wheel_RotAcc[rad/s**2]"
  __TDD__FrontRight_Tire_DynamicRadius[m]/1 -> FrontRight_Tire_DynamicRadius[m]___UNIQUE_1/1  "FrontRight_Tire_DynamicRadius[m]"
  __TDD__RearLeft_Tire_LongSpd(ContactSys)[m/s]/1 -> RearLeft_Tire_LongSpd(ContactSys)[m/s]___UNIQUE_1/1  "RearLeft_Tire_LongSpd(ContactSys)[m/s]"
  __TDD__RearLeft_Wheel_RotSpd[rad/s]/1 -> RearLeft_Wheel_RotSpd[rad/s]___UNIQUE_1/1  "RearLeft_Wheel_RotSpd[rad/s]"
  __TDD__RearLeft_Wheel_RotAcc[rad/s**2]/1 -> RearLeft_Wheel_RotAcc[rad/s**2]___UNIQUE_1/1  "RearLeft_Wheel_RotAcc[rad/s**2]"
  __TDD__RearLeft_Tire_DynamicRadius[m]/1 -> RearLeft_Tire_DynamicRadius[m]___UNIQUE_1/1  "RearLeft_Tire_DynamicRadius[m]"
  __TDD__RearRight_Tire_LongSpd(ContactSys)[m/s]/1 -> RearRight_Tire_LongSpd(ContactSys)[m/s]___UNIQUE_1/1  "RearRight_Tire_LongSpd(ContactSys)[m/s]"
  __TDD__RearRight_Wheel_RotSpd[rad/s]/1 -> RearRight_Wheel_RotSpd[rad/s]___UNIQUE_1/1  "RearRight_Wheel_RotSpd[rad/s]"
  __TDD__RearRight_Wheel_RotAcc[rad/s**2]/1 -> RearRight_Wheel_RotAcc[rad/s**2]___UNIQUE_1/1  "RearRight_Wheel_RotAcc[rad/s**2]"
  __TDD__RearRight_Tire_DynamicRadius[m]/1 -> RearRight_Tire_DynamicRadius[m]___UNIQUE_1/1  "RearRight_Tire_DynamicRadius[m]"
  __TDD__FrontLeft_Tire_UnloadedRadius[m]/1 -> FrontLeft_Tire_UnloadedRadius[m]___UNIQUE_1/1  "FrontLeft_Tire_UnloadedRadius[m]"
  __TDD__RearLeft_Tire_UnloadedRadius[m]/1 -> RearLeft_Tire_UnloadedRadius[m]___UNIQUE_1/1  "RearLeft_Tire_UnloadedRadius[m]"
  __TDD__FrontLeft_Wheel_BrakeTrqPressRatio[m**3]/1 -> FrontLeft_Wheel_BrakeTrqPressRatio[m**3]___UNIQUE_1/1  "FrontLeft_Wheel_BrakeTrqPressRatio[m**3]"
  __TDD__RearLeft_Wheel_BrakeTrqPressRatio[m**3]/1 -> RearLeft_Wheel_BrakeTrqPressRatio[m**3]___UNIQUE_1/1  "RearLeft_Wheel_BrakeTrqPressRatio[m**3]"

== system PassengerCar/Vehicle/Drivetrain/DrivetrainPhysics/DrivetrainPhysicsInputs/InputFromAuxiliaries ==
  fromAuxiliaries : Inport
  TDBusSelector : BusSelector  OutputSignals=StarterInrt[kgm**2],StarterTrq[Nm]
  __TDD__StarterInrt[kgm**2] : Demux  Outputs=[1]
  __TDD__StarterTrq[Nm] : Demux  Outputs=[1]
  StarterInrt[kgm**2]___UNIQUE_1 : Outport  Description=|  PortDimensions=[1]  VectorParamsAs1DForOutWhenUnconnected=off
      | <name>StarterInrt[kgm**2]</name>
      | <comment></comment>
  StarterTrq[Nm]___UNIQUE_1 : Outport  Description=|  Port=2  PortDimensions=[1]  VectorParamsAs1DForOutWhenUnconnected=off
      | <name>StarterTrq[Nm]</name>
      | <comment></comment>
  wires:
  fromAuxiliaries/1 -> TDBusSelector/1
  TDBusSelector/1 -> __TDD__StarterInrt[kgm**2]/1  "<StarterInrt[kgm**2]>"
  TDBusSelector/2 -> __TDD__StarterTrq[Nm]/1  "<StarterTrq[Nm]>"
  __TDD__StarterInrt[kgm**2]/1 -> StarterInrt[kgm**2]___UNIQUE_1/1  "StarterInrt[kgm**2]"
  __TDD__StarterTrq[Nm]/1 -> StarterTrq[Nm]___UNIQUE_1/1  "StarterTrq[Nm]"

== system PassengerCar/Vehicle/Drivetrain/DrivetrainPhysics/DrivetrainPhysicsInputs/InputFromCTRL ==
  fromCTRL : Inport
  TDBusSelector : BusSelector  OutputSignals=CTRL.LongitudinalControl.InitialEngineSpeed[rad/s],CTRL.LongitudinalControl.InitialGear[-4;20],CTRL.LongitudinalControl.ClutchPos[0_1],CTRL.LongitudinalControl.ManualGear[-4;20],CTRL.LongitudinalControl.TransferCaseLock[0;1],CTRL.LongitudinalControl.FrontDifferentialLock[0;1],CTRL.LongitudinalControl.RearDifferentialLock[0;1],CTRL.LongitudinalControl.Rear2DifferentialLock[0;1],CTRL.LongitudinalControl.Rear3DifferentialLock[0;1],CTRL.TemperatureControl.TransmissionTemp[K],CTRL.TemperatureControl.TransferCaseTemp[K],CTRL.TemperatureControl.FrontDifferentialTemp[K],CTRL.TemperatureControl.RearDifferentialTemp[K],CTRL.TemperatureControl.Rear2DifferentialTemp[K],CTRL.TemperatureControl.Rear3DifferentialTemp[K]
  __TDD__ClutchPos[0_1] : Demux  Outputs=[1]
  __TDD__FrontDifferentialLock[0;1] : Demux  Outputs=[1]
  __TDD__FrontDifferentialTemp[K] : Demux  Outputs=[1]
  __TDD__InitialEngineSpeed[rad/s] : Demux  Outputs=[1]
  __TDD__InitialGear[-4;20] : Demux  Outputs=[1]
  __TDD__ManualGear[-4;20] : Demux  Outputs=[1]
  __TDD__Rear2DifferentialLock[0;1] : Demux  Outputs=[1]
  __TDD__Rear2DifferentialTemp[K] : Demux  Outputs=[1]
  __TDD__Rear3DifferentialLock[0;1] : Demux  Outputs=[1]
  __TDD__Rear3DifferentialTemp[K] : Demux  Outputs=[1]
  __TDD__RearDifferentialLock[0;1] : Demux  Outputs=[1]
  __TDD__RearDifferentialTemp[K] : Demux  Outputs=[1]
  __TDD__TransferCaseLock[0;1] : Demux  Outputs=[1]
  __TDD__TransferCaseTemp[K] : Demux  Outputs=[1]
  __TDD__TransmissionTemp[K] : Demux  Outputs=[1]
  InitialEngineSpeed[rad/s]___UNIQUE_1 : Outport  Description=|  PortDimensions=[1]  VectorParamsAs1DForOutWhenUnconnected=off
      | <name>CTRL.LongitudinalControl.InitialEngineSpeed[rad/s]</name>
      | <comment></comment>
  InitialGear[-4;20]___UNIQUE_1 : Outport  Description=|  Port=2  PortDimensions=[1]  VectorParamsAs1DForOutWhenUnconnected=off
      | <name>CTRL.LongitudinalControl.InitialGear[-4;20]</name>
      | <comment></comment>
  ClutchPos[0_1]___UNIQUE_1 : Outport  Description=|  Port=3  PortDimensions=[1]  VectorParamsAs1DForOutWhenUnconnected=off
      | <name>CTRL.LongitudinalControl.ClutchPos[0_1]</name>
      | <comment></comment>
  ManualGear[-4;20]___UNIQUE_1 : Outport  Description=|  Port=4  PortDimensions=[1]  VectorParamsAs1DForOutWhenUnconnected=off
      | <name>CTRL.LongitudinalControl.ManualGear[-4;20]</name>
      | <comment></comment>
  TransferCaseLock[0;1]___UNIQUE_1 : Outport  Description=|  Port=5  PortDimensions=[1]  VectorParamsAs1DForOutWhenUnconnected=off
      | <name>CTRL.LongitudinalControl.TransferCaseLock[0;1]</name>
      | <comment></comment>
  FrontDifferentialLock[0;1]___UNIQUE_1 : Outport  Description=|  Port=6  PortDimensions=[1]  VectorParamsAs1DForOutWhenUnconnected=off
      | <name>CTRL.LongitudinalControl.FrontDifferentialLock[0;1]</name>
      | <comment></comment>
  RearDifferentialLock[0;1]___UNIQUE_1 : Outport  Description=|  Port=7  PortDimensions=[1]  VectorParamsAs1DForOutWhenUnconnected=off
      | <name>CTRL.LongitudinalControl.RearDifferentialLock[0;1]</name>
      | <comment></comment>
  Rear2DifferentialLock[0;1]___UNIQUE_1 : Outport  Description=|  Port=8  PortDimensions=[1]  VectorParamsAs1DForOutWhenUnconnected=off
      | <name>CTRL.LongitudinalControl.Rear2DifferentialLock[0;1]</name>
      | <comment></comment>
  Rear3DifferentialLock[0;1]___UNIQUE_1 : Outport  Description=|  Port=9  PortDimensions=[1]  VectorParamsAs1DForOutWhenUnconnected=off
      | <name>CTRL.LongitudinalControl.Rear3DifferentialLock[0;1]</name>
      | <comment></comment>
  TransmissionTemp[K]___UNIQUE_1 : Outport  Description=|  Port=10  PortDimensions=[1]  VectorParamsAs1DForOutWhenUnconnected=off
      | <name>CTRL.TemperatureControl.TransmissionTemp[K]</name>
      | <comment></comment>
  TransferCaseTemp[K]___UNIQUE_1 : Outport  Description=|  Port=11  PortDimensions=[1]  VectorParamsAs1DForOutWhenUnconnected=off
      | <name>CTRL.TemperatureControl.TransferCaseTemp[K]</name>
      | <comment></comment>
  FrontDifferentialTemp[K]___UNIQUE_1 : Outport  Description=|  Port=12  PortDimensions=[1]  VectorParamsAs1DForOutWhenUnconnected=off
      | <name>CTRL.TemperatureControl.FrontDifferentialTemp[K]</name>
      | <comment></comment>
  RearDifferentialTemp[K]___UNIQUE_1 : Outport  Description=|  Port=13  PortDimensions=[1]  VectorParamsAs1DForOutWhenUnconnected=off
      | <name>CTRL.TemperatureControl.RearDifferentialTemp[K]</name>
      | <comment></comment>
  Rear2DifferentialTemp[K]___UNIQUE_1 : Outport  Description=|  Port=14  PortDimensions=[1]  VectorParamsAs1DForOutWhenUnconnected=off
      | <name>CTRL.TemperatureControl.Rear2DifferentialTemp[K]</name>
      | <comment></comment>
  Rear3DifferentialTemp[K]___UNIQUE_1 : Outport  Description=|  Port=15  PortDimensions=[1]  VectorParamsAs1DForOutWhenUnconnected=off
      | <name>CTRL.TemperatureControl.Rear3DifferentialTemp[K]</name>
      | <comment></comment>
  wires:
  fromCTRL/1 -> TDBusSelector/1
  TDBusSelector/1 -> __TDD__InitialEngineSpeed[rad/s]/1  "<InitialEngineSpeed[rad/s]>"
  TDBusSelector/2 -> __TDD__InitialGear[-4;20]/1  "<InitialGear[-4;20]>"
  TDBusSelector/3 -> __TDD__ClutchPos[0_1]/1  "<ClutchPos[0_1]>"
  TDBusSelector/4 -> __TDD__ManualGear[-4;20]/1  "<ManualGear[-4;20]>"
  TDBusSelector/5 -> __TDD__TransferCaseLock[0;1]/1  "<TransferCaseLock[0;1]>"
  TDBusSelector/6 -> __TDD__FrontDifferentialLock[0;1]/1  "<FrontDifferentialLock[0;1]>"
  TDBusSelector/7 -> __TDD__RearDifferentialLock[0;1]/1  "<RearDifferentialLock[0;1]>"
  TDBusSelector/8 -> __TDD__Rear2DifferentialLock[0;1]/1  "<Rear2DifferentialLock[0;1]>"
  TDBusSelector/9 -> __TDD__Rear3DifferentialLock[0;1]/1  "<Rear3DifferentialLock[0;1]>"
  TDBusSelector/10 -> __TDD__TransmissionTemp[K]/1  "<TransmissionTemp[K]>"
  TDBusSelector/11 -> __TDD__TransferCaseTemp[K]/1  "<TransferCaseTemp[K]>"
  TDBusSelector/12 -> __TDD__FrontDifferentialTemp[K]/1  "<FrontDifferentialTemp[K]>"
  TDBusSelector/13 -> __TDD__RearDifferentialTemp[K]/1  "<RearDifferentialTemp[K]>"
  TDBusSelector/14 -> __TDD__Rear2DifferentialTemp[K]/1  "<Rear2DifferentialTemp[K]>"
  TDBusSelector/15 -> __TDD__Rear3DifferentialTemp[K]/1  "<Rear3DifferentialTemp[K]>"
  __TDD__InitialEngineSpeed[rad/s]/1 -> InitialEngineSpeed[rad/s]___UNIQUE_1/1  "InitialEngineSpeed[rad/s]"
  __TDD__InitialGear[-4;20]/1 -> InitialGear[-4;20]___UNIQUE_1/1  "InitialGear[-4;20]"
  __TDD__ClutchPos[0_1]/1 -> ClutchPos[0_1]___UNIQUE_1/1  "ClutchPos[0_1]"
  __TDD__ManualGear[-4;20]/1 -> ManualGear[-4;20]___UNIQUE_1/1  "ManualGear[-4;20]"
  __TDD__TransferCaseLock[0;1]/1 -> TransferCaseLock[0;1]___UNIQUE_1/1  "TransferCaseLock[0;1]"
  __TDD__FrontDifferentialLock[0;1]/1 -> FrontDifferentialLock[0;1]___UNIQUE_1/1  "FrontDifferentialLock[0;1]"
  __TDD__RearDifferentialLock[0;1]/1 -> RearDifferentialLock[0;1]___UNIQUE_1/1  "RearDifferentialLock[0;1]"
  __TDD__Rear2DifferentialLock[0;1]/1 -> Rear2DifferentialLock[0;1]___UNIQUE_1/1  "Rear2DifferentialLock[0;1]"
  __TDD__Rear3DifferentialLock[0;1]/1 -> Rear3DifferentialLock[0;1]___UNIQUE_1/1  "Rear3DifferentialLock[0;1]"
  __TDD__TransmissionTemp[K]/1 -> TransmissionTemp[K]___UNIQUE_1/1  "TransmissionTemp[K]"
  __TDD__TransferCaseTemp[K]/1 -> TransferCaseTemp[K]___UNIQUE_1/1  "TransferCaseTemp[K]"
  __TDD__FrontDifferentialTemp[K]/1 -> FrontDifferentialTemp[K]___UNIQUE_1/1  "FrontDifferentialTemp[K]"
  __TDD__RearDifferentialTemp[K]/1 -> RearDifferentialTemp[K]___UNIQUE_1/1  "RearDifferentialTemp[K]"
  __TDD__Rear2DifferentialTemp[K]/1 -> Rear2DifferentialTemp[K]___UNIQUE_1/1  "Rear2DifferentialTemp[K]"
  __TDD__Rear3DifferentialTemp[K]/1 -> Rear3DifferentialTemp[K]___UNIQUE_1/1  "Rear3DifferentialTemp[K]"

== system PassengerCar/Vehicle/Drivetrain/DrivetrainPhysics/DrivetrainPhysicsInputs/InputFromDrivetrainControlUnit ==
  fromDrivetrainControlUnit : Inport
  TDBusSelector : BusSelector  OutputSignals=TransmissionControlUnit.AutomatedManualClutchPos[0_1],TransmissionControlUnit.LockUpClutchPos[0_1],TransmissionControlUnit.Gear[-4;20]
  __TDD__AutomatedManualClutchPos[0_1] : Demux  Outputs=[1]
  __TDD__AutomaticGear[-4;20] : Demux  Outputs=[1]
  __TDD__LockUpClutchPos[0_1] : Demux  Outputs=[1]
  AutomatedManualClutchPos[0_1]___UNIQUE_1 : Outport  Description=|  PortDimensions=[1]  VectorParamsAs1DForOutWhenUnconnected=off
      | <name>TransmissionControlUnit.AutomatedManualClutchPos[0_1]</name>
      | <comment></comment>
  LockUpClutchPos[0_1]___UNIQUE_1 : Outport  Description=|  Port=2  PortDimensions=[1]  VectorParamsAs1DForOutWhenUnconnected=off
      | <name>TransmissionControlUnit.LockUpClutchPos[0_1]</name>
      | <comment></comment>
  AutomaticGear[-4;20]___UNIQUE_1 : Outport  Description=|  Port=3  PortDimensions=[1]  VectorParamsAs1DForOutWhenUnconnected=off
      | <name>TransmissionControlUnit.Gear[-4;20]</name>
      | <comment></comment>
  wires:
  fromDrivetrainControlUnit/1 -> TDBusSelector/1
  TDBusSelector/1 -> __TDD__AutomatedManualClutchPos[0_1]/1  "<AutomatedManualClutchPos[0_1]>"
  TDBusSelector/2 -> __TDD__LockUpClutchPos[0_1]/1  "<LockUpClutchPos[0_1]>"
  TDBusSelector/3 -> __TDD__AutomaticGear[-4;20]/1  "<Gear[-4;20]>"
  __TDD__AutomatedManualClutchPos[0_1]/1 -> AutomatedManualClutchPos[0_1]___UNIQUE_1/1  "AutomatedManualClutchPos[0_1]"
  __TDD__LockUpClutchPos[0_1]/1 -> LockUpClutchPos[0_1]___UNIQUE_1/1  "LockUpClutchPos[0_1]"
  __TDD__AutomaticGear[-4;20]/1 -> AutomaticGear[-4;20]___UNIQUE_1/1  "AutomaticGear[-4;20]"

== system PassengerCar/Vehicle/Drivetrain/DrivetrainPhysics/DrivetrainPhysicsInputs/InputFromEngine ==
  fromEngine : Inport
  TDBusSelector : BusSelector  OutputSignals=EnginePhysics.Mechanics.EngInrt[kg*m**2],EnginePhysics.Mechanics.EngTrq[Nm],EnginePhysics.Mechanics.DerivativeOfEngTrq_wrt_CrankAng[Nm/rad],EnginePhysics.Mechanics.DerivativeOfEngTrq_wrt_EngSpd[Nm/(rad/s)],EnginePhysics.Mechanics.MeanEngFrictionTrq[Nm],EngineControlUnit.EngIdleSpd[rad/s]
  __TDD__DerivativeOfEngTrq_wrt_CrankAng[Nm/rad] : Demux  Outputs=[1]
  __TDD__DerivativeOfEngTrq_wrt_EngSpd[Nm/(rad/s)] : Demux  Outputs=[1]
  __TDD__EngIdleSpd[rad/s] : Demux  Outputs=[1]
  __TDD__EngInrt[kg*m**2] : Demux  Outputs=[1]
  __TDD__EngTrq[Nm] : Demux  Outputs=[1]
  __TDD__MeanEngFrictionTrq[Nm] : Demux  Outputs=[1]
  EngInrt[kg*m**2]___UNIQUE_1 : Outport  Description=|  PortDimensions=[1]  VectorParamsAs1DForOutWhenUnconnected=off
      | <name>EnginePhysics.Mechanics.EngInrt[kg*m**2]</name>
      | <comment></comment>
  EngTrq[Nm]___UNIQUE_1 : Outport  Description=|  Port=2  PortDimensions=[1]  VectorParamsAs1DForOutWhenUnconnected=off
      | <name>EnginePhysics.Mechanics.EngTrq[Nm]</name>
      | <comment></comment>
  DerivativeOfEngTrq_wrt_CrankAng[Nm/rad]___UNIQUE_1 : Outport  Description=|  Port=3  PortDimensions=[1]  VectorParamsAs1DForOutWhenUnconnected=off
      | <name>EnginePhysics.Mechanics.DerivativeOfEngTrq_wrt_CrankAng[Nm/rad]</name>
      | <comment></comment>
  DerivativeOfEngTrq_wrt_EngSpd[Nm/(rad/s)]___UNIQUE_1 : Outport  Description=|  Port=4  PortDimensions=[1]  VectorParamsAs1DForOutWhenUnconnected=off
      | <name>EnginePhysics.Mechanics.DerivativeOfEngTrq_wrt_EngSpd[Nm/(rad/s)]</name>
      | <comment></comment>
  MeanEngFrictionTrq[Nm]___UNIQUE_1 : Outport  Description=|  Port=5  PortDimensions=[1]  VectorParamsAs1DForOutWhenUnconnected=off
      | <name>EnginePhysics.Mechanics.MeanEngFrictionTrq[Nm]</name>
      | <comment></comment>
  EngIdleSpd[rad/s]___UNIQUE_1 : Outport  Description=|  Port=6  PortDimensions=[1]  VectorParamsAs1DForOutWhenUnconnected=off
      | <name>EngineControlUnit.EngIdleSpd[rad/s]</name>
      | <comment></comment>
  wires:
  fromEngine/1 -> TDBusSelector/1
  TDBusSelector/1 -> __TDD__EngInrt[kg*m**2]/1  "<EngInrt[kg*m**2]>"
  TDBusSelector/2 -> __TDD__EngTrq[Nm]/1  "<EngTrq[Nm]>"
  TDBusSelector/3 -> __TDD__DerivativeOfEngTrq_wrt_CrankAng[Nm/rad]/1  "<DerivativeOfEngTrq_wrt_CrankAng[Nm/rad]>"
  TDBusSelector/4 -> __TDD__DerivativeOfEngTrq_wrt_EngSpd[Nm/(rad/s)]/1  "<DerivativeOfEngTrq_wrt_EngSpd[Nm/(rad/s)]>"
  TDBusSelector/5 -> __TDD__MeanEngFrictionTrq[Nm]/1  "<MeanEngFrictionTrq[Nm]>"
  TDBusSelector/6 -> __TDD__EngIdleSpd[rad/s]/1  "<EngIdleSpd[rad/s]>"
  __TDD__EngInrt[kg*m**2]/1 -> EngInrt[kg*m**2]___UNIQUE_1/1  "EngInrt[kg*m**2]"
  __TDD__EngTrq[Nm]/1 -> EngTrq[Nm]___UNIQUE_1/1  "EngTrq[Nm]"
  __TDD__DerivativeOfEngTrq_wrt_CrankAng[Nm/rad]/1 -> DerivativeOfEngTrq_wrt_CrankAng[Nm/rad]___UNIQUE_1/1  "DerivativeOfEngTrq_wrt_CrankAng[Nm/rad]"
  __TDD__DerivativeOfEngTrq_wrt_EngSpd[Nm/(rad/s)]/1 -> DerivativeOfEngTrq_wrt_EngSpd[Nm/(rad/s)]___UNIQUE_1/1  "DerivativeOfEngTrq_wrt_EngSpd[Nm/(rad/s)]"
  __TDD__MeanEngFrictionTrq[Nm]/1 -> MeanEngFrictionTrq[Nm]___UNIQUE_1/1  "MeanEngFrictionTrq[Nm]"
  __TDD__EngIdleSpd[rad/s]/1 -> EngIdleSpd[rad/s]___UNIQUE_1/1  "EngIdleSpd[rad/s]"
